simulink model "level1_newPlant"  (R2023b)
settings: Solver=ode4  StartTime=0.0  StopTime=600  FixedStep=1e-2  RelTol=1e-3
settings Model: Creator=evreng  LastModifiedBy=evreng

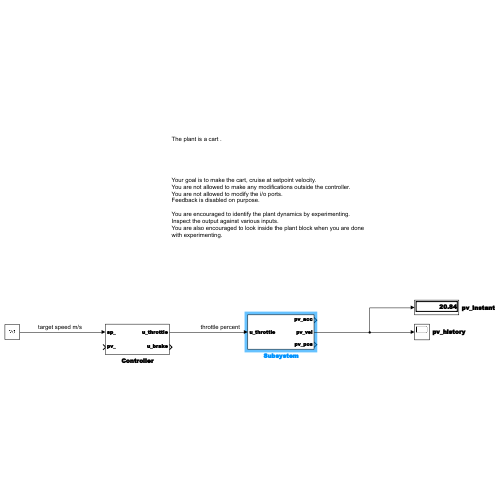
[thumbnail: Simulink's stored preview of the top-level diagram]
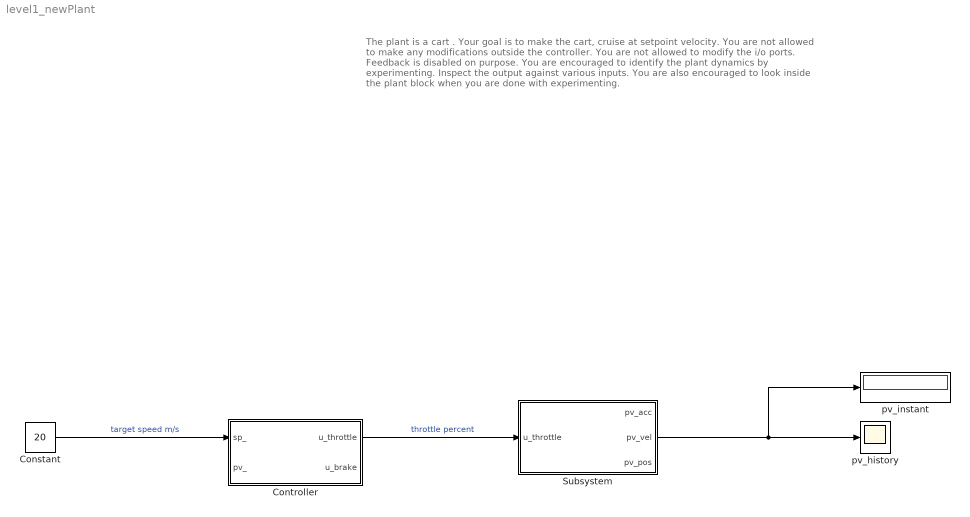
== system level1_newPlant ==
  note: The plant is a cart .
      |
      |
      |
      |
      |
      | Your goal is to make the cart, cruise at setpoint velocity.
      | You are not allowed to make any modifications outside the controller.
      | You are not allowed to modify the i/o ports.
      | Feedback is disabled on purpose.
      |
      | You are encouraged to identify the plant dynamics by experimenting. Inspect the output against various inputs.
      | You are also encouraged to look inside the plant block when you are done with experimenting.
  Constant : Constant  Value=20
  Controller : Subsystem
  Subsystem : Subsystem
  pv_history : Scope
  pv_instant : Display
  wires:
  Controller/1(u_throttle) -> Subsystem/1(u_throttle)  "throttle percent"
  Constant/1 -> Controller/1(sp_)  "target speed m/s"
  Subsystem/2(pv_vel) -> pv_history/1, pv_instant/1

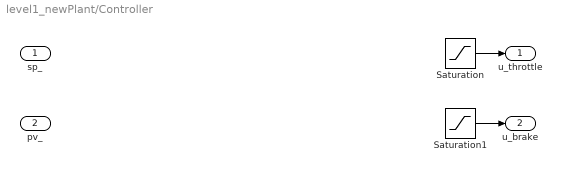
== system level1_newPlant/Controller ==
  sp_ : Inport
  pv_ : Inport  Port=2
  Saturation : Saturate  UpperLimit=1  LowerLimit=0
  Saturation1 : Saturate  UpperLimit=1  LowerLimit=0
  u_throttle : Outport
  u_brake : Outport  Port=2
  wires:
  Saturation/1 -> u_throttle/1
  Saturation1/1 -> u_brake/1

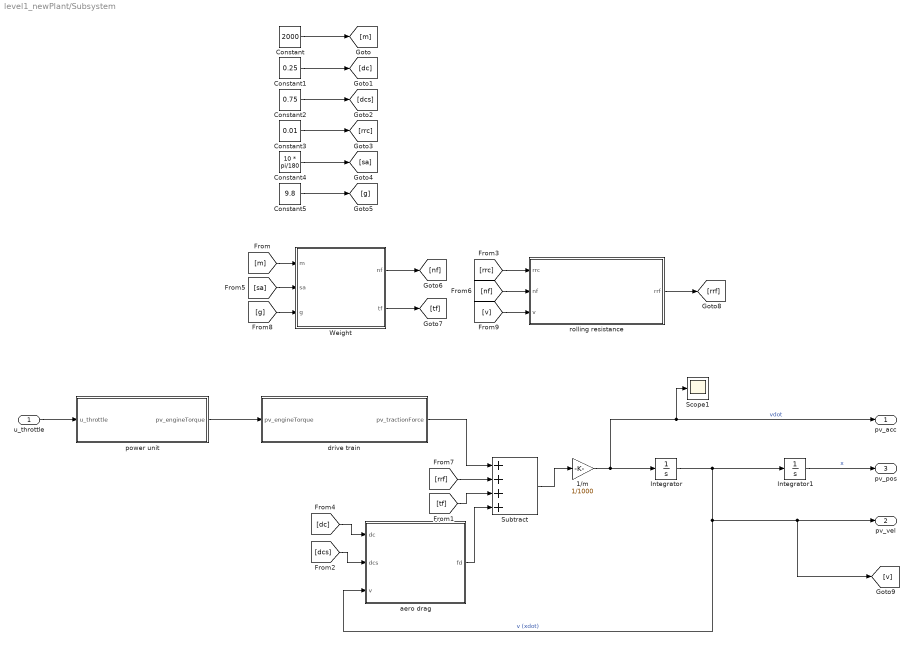
== system level1_newPlant/Subsystem ==
  u_throttle : Inport
  1/m : Gain  Gain=1/1000
  Constant : Constant  Value=2000
  Constant1 : Constant  Value=0.25
  Constant2 : Constant  Value=0.75
  Constant3 : Constant  Value=0.01
  Constant4 : Constant  Value=10 * pi/180
  Constant5 : Constant  Value=9.8
  Integrator : Integrator
  Integrator1 : Integrator
  Scope1 : Scope
  Subtract : Sum  Inputs=++++
  Weight : MATLAB Function  TreatAsAtomicUnit=on
  aero drag : MATLAB Function  TreatAsAtomicUnit=on
  drive train : Subsystem
  power unit : Subsystem
  rolling resistance : MATLAB Function  TreatAsAtomicUnit=on
  pv_acc : Outport
  pv_vel : Outport  Port=2
  pv_pos : Outport  Port=3
  wires:
  [v] -> rolling resistance/3(v)
  [m] -> Weight/1(m)
  Constant/1 -> [m]
  u_throttle/1 -> power unit/1(u_throttle)
  [g] -> Weight/3(g)
  Constant3/1 -> [rrc]
  [dc] -> aero drag/1(dc)
  [tf] -> Subtract/3
  1/m/1 -> Integrator/1, pv_acc/1, Scope1/1  "vdot"
  [nf] -> rolling resistance/2(nf)
  [sa] -> Weight/2(sa)
  Weight/1(nf) -> [nf]
  Constant2/1 -> [dcs]
  Weight/2(tf) -> [tf]
  Integrator1/1 -> pv_pos/1  "x"
  drive train/1(pv_tractionForce) -> Subtract/1
  Constant5/1 -> [g]
  rolling resistance/1(rrf) -> [rrf]
  aero drag/1(fd) -> Subtract/4
  Subtract/1 -> 1/m/1
  Constant1/1 -> [dc]
  Constant4/1 -> [sa]
  [rrc] -> rolling resistance/1(rrc)
  Integrator/1 -> aero drag/3(v), pv_vel/1, [v], Integrator1/1  "v (xdot)"
  [dcs] -> aero drag/2(dcs)
  [rrf] -> Subtract/2
  power unit/1(pv_engineTorque) -> drive train/1(pv_engineTorque)

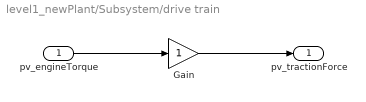
== system level1_newPlant/Subsystem/drive train ==
  pv_engineTorque : Inport
  Gain : Gain
  pv_tractionForce : Outport
  wires:
  pv_engineTorque/1 -> Gain/1
  Gain/1 -> pv_tractionForce/1

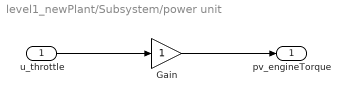
== system level1_newPlant/Subsystem/power unit ==
  u_throttle : Inport
  Gain : Gain
  pv_engineTorque : Outport
  wires:
  u_throttle/1 -> Gain/1
  Gain/1 -> pv_engineTorque/1

== matlab function level1_newPlant/Subsystem/rolling resistance ==
  data: rrc input; rrf output; nf input; v input
function rrf = rollingResistance(rrc, nf, v)
tol = 1e-3;
if abs(v) > tol
    rrf = rrc * nf * (-1 * sign(v));
else
    rrf = 0;
end

== matlab function level1_newPlant/Subsystem/aero drag ==
  data: dc input; fd output; dcs input; v input
function fd = aeroDrag(dc, dcs, v)
fd = 0.5 * dc * dcs * v ^ 2 * (-1 * sign(v));

== matlab function level1_newPlant/Subsystem/Weight ==
  data: m input; nf output; sa input; tf output; g input
function [nf, tf] = fcn(m, sa, g)
nf = m * g * cos(sa);
tf = -1 * m * g * sin(sa);
